simulink model "BD_PAR_AUTO_base_model"  (Simulink 10.3)
settings: Solver=ode1  StartTime=0.0  StopTime=max(cyc_mph(:,1))  FixedStep=1  MaxStep=1  RelTol=1e-3  AbsTol=1e-3
undefined symbols (not defined in the file): acc_dcdc_eff, acc_elec_eff, acc_elec_pwr, acc_mech_eff, acc_mech_pwr, acc_mech_trq, air_cp, amb_tmp, cs_charge_deplete_bool, cs_charge_trq, cs_electric_decel_spd, cs_electric_launch_spd_hi, cs_electric_launch_spd_lo, cs_hi_soc, cs_lo_soc, cs_min_trq_frac, cs_off_trq_frac, cyc_avg_time, cyc_cargo_mass, cyc_elevation_init, cyc_filter_bool, cyc_grade, cyc_mph, enable_sim_stop_distance, enable_sim_stop_max_spd, enable_sim_stop_speed, enable_sim_stop_time, enable_stop, enable_stop_fc, ess_cap_scale, ess_coulombic_eff, ess_init_soc, ess_max_ah_cap, ess_max_volts, ess_min_volts, ess_mod_airflow, ess_mod_cp, ess_mod_init_tmp, ess_module_mass, ess_module_num, ess_on, ess_r_chg, ess_r_dis, ess_res_scale_coef, ess_res_scale_fun, ess_set_tmp, ess_soc, ess_th_calc, ess_th_res_off, ess_th_res_on, ess_tmp, ess_voc, ex_calc, ex_cat_co_frac, ex_cat_ext_cp, ex_cat_ext_emisv, ex_cat_ext_init_tmp, ex_cat_ext_mass, ex_cat_ext_sarea, ex_cat_hc_frac ... (+168)
(part 9 of 15)

== system BD_PAR_AUTO_base_model/electric acc loads <acc>/Electrical Accessory Loads v2 <acc>/backward model/electrical accessories (W)/Electrical Accessories: Time Variable/Elec Aux Loads 14V Pwr/Engine ==
  Average Watts : Constant  Value=vinf.AuxLoads.Engine.AverageWatts
  Memory : Memory
  On : Constant  Value=vinf.AuxLoads.Engine.On
  Product : Product  Inputs=4  InputSameDT=on  RndMeth=Zero  SaturateOnIntegerOverflow=on  OutDataTypeStr=Inherit: Same as first input
  Out1 : Outport
  wires:
  Average Watts/1 -> Product/4
  Product/1 -> Out1/1
  On/1 -> Product/1
  [key_on] -> Product/3
  [engine_on] -> Memory/1
  Memory/1 -> Product/2

== system BD_PAR_AUTO_base_model/electric acc loads <acc>/Electrical Accessory Loads v2 <acc>/backward model/electrical accessories (W)/Electrical Accessories: Time Variable/Elec Aux Loads 14V Pwr/ExternalLights ==
  Average Watts : Constant  Value=vinf.AuxLoads.ExternalLights.AverageWatts
  On : Constant  Value=vinf.AuxLoads.ExternalLights.On
  Product : Product  Inputs=3  InputSameDT=on  RndMeth=Zero  SaturateOnIntegerOverflow=on  OutDataTypeStr=Inherit: Same as first input
  Subsystem : Subsystem  mask{ModelName='ExternalLights'}
      mask prompts: ModelName "Load Name (example: 'Radio')"
  Out1 : Outport
  wires:
  Product/1 -> Out1/1
  Subsystem/1(On/Off Control) -> Product/2
  On/1 -> Product/1
  Average Watts/1 -> Product/3

== system BD_PAR_AUTO_base_model/electric acc loads <acc>/Electrical Accessory Loads v2 <acc>/backward model/electrical accessories (W)/Electrical Accessories: Time Variable/Elec Aux Loads 14V Pwr/FrontHVAC ==
  Average Watts : Constant  Value=vinf.AuxLoads.FrontHVAC.AverageWatts
  On : Constant  Value=vinf.AuxLoads.FrontHVAC.On
  Product : Product  Inputs=3  InputSameDT=on  RndMeth=Zero  SaturateOnIntegerOverflow=on  OutDataTypeStr=Inherit: Same as first input
  Subsystem : Subsystem  mask{ModelName='FrontHVAC'}
      mask prompts: ModelName "Load Name (example: 'Radio')"
  Out1 : Outport
  wires:
  Product/1 -> Out1/1
  Subsystem/1(On/Off Control) -> Product/2
  On/1 -> Product/1
  Average Watts/1 -> Product/3

== system BD_PAR_AUTO_base_model/electric acc loads <acc>/Electrical Accessory Loads v2 <acc>/backward model/electrical accessories (W)/Electrical Accessories: Time Variable/Elec Aux Loads 14V Pwr/FrontWipers ==
  Average Watts : Constant  Value=vinf.AuxLoads.FrontWipers.AverageWatts
  On : Constant  Value=vinf.AuxLoads.FrontWipers.On
  Product : Product  Inputs=3  InputSameDT=on  RndMeth=Zero  SaturateOnIntegerOverflow=on  OutDataTypeStr=Inherit: Same as first input
  Subsystem : Subsystem  mask{ModelName='FrontWipers'}
      mask prompts: ModelName "Load Name (example: 'Radio')"
  Out1 : Outport
  wires:
  Product/1 -> Out1/1
  Subsystem/1(On/Off Control) -> Product/2
  On/1 -> Product/1
  Average Watts/1 -> Product/3

== system BD_PAR_AUTO_base_model/electric acc loads <acc>/Electrical Accessory Loads v2 <acc>/backward model/electrical accessories (W)/Electrical Accessories: Time Variable/Elec Aux Loads 14V Pwr/HeatedSeats ==
  Average Watts : Constant  Value=vinf.AuxLoads.HeatedSeats.AverageWatts
  Num : Constant  Value=vinf.AuxLoads.HeatedSeats.Num
  On : Constant  Value=vinf.AuxLoads.HeatedSeats.On
  Product : Product  Inputs=4  InputSameDT=on  RndMeth=Zero  SaturateOnIntegerOverflow=on  OutDataTypeStr=Inherit: Same as first input
  Subsystem : Subsystem  mask{ModelName='HeatedSeats'}
      mask prompts: ModelName "Load Name (example: 'Radio')"
  Out1 : Outport
  wires:
  Num/1 -> Product/2
  On/1 -> Product/1
  Average Watts/1 -> Product/4
  Product/1 -> Out1/1
  Subsystem/1(On/Off Control) -> Product/3

== system BD_PAR_AUTO_base_model/electric acc loads <acc>/Electrical Accessory Loads v2 <acc>/backward model/electrical accessories (W)/Electrical Accessories: Time Variable/Elec Aux Loads 14V Pwr/Misc ==
  Average Watts : Constant  Value=vinf.AuxLoads.Misc.AverageWatts
  On : Constant  Value=vinf.AuxLoads.Misc.On
  Product : Product  Inputs=3  InputSameDT=on  RndMeth=Zero  SaturateOnIntegerOverflow=on  OutDataTypeStr=Inherit: Same as first input
  Out1 : Outport
  wires:
  Product/1 -> Out1/1
  On/1 -> Product/1
  [key_on] -> Product/2
  Average Watts/1 -> Product/3

== system BD_PAR_AUTO_base_model/electric acc loads <acc>/Electrical Accessory Loads v2 <acc>/backward model/electrical accessories (W)/Electrical Accessories: Time Variable/Elec Aux Loads 14V Pwr/RadiatorCoolingFan ==
  Average Watts : Constant  Value=vinf.AuxLoads.RadiatorCoolingFan.AverageWatts
  On : Constant  Value=vinf.AuxLoads.RadiatorCoolingFan.On
  Product : Product  Inputs=3  InputSameDT=on  RndMeth=Zero  SaturateOnIntegerOverflow=on  OutDataTypeStr=Inherit: Same as first input
  Subsystem : Subsystem  mask{ModelName='RadiatorCoolingFan'}
      mask prompts: ModelName "Load Name (example: 'Radio')"
  Out1 : Outport
  wires:
  Product/1 -> Out1/1
  Subsystem/1(On/Off Control) -> Product/2
  On/1 -> Product/1
  Average Watts/1 -> Product/3

== system BD_PAR_AUTO_base_model/electric acc loads <acc>/Electrical Accessory Loads v2 <acc>/backward model/electrical accessories (W)/Electrical Accessories: Time Variable/Elec Aux Loads 14V Pwr/Radio ==
  Average Watts : Constant  Value=vinf.AuxLoads.Radio.AverageWatts
  Num : Constant  Value=vinf.AuxLoads.Radio.Num
  On : Constant  Value=vinf.AuxLoads.Radio.On
  Product : Product  Inputs=4  InputSameDT=on  RndMeth=Zero  SaturateOnIntegerOverflow=on  OutDataTypeStr=Inherit: Same as first input
  Subsystem : Subsystem  mask{ModelName='Radio'}
      mask prompts: ModelName "Load Name (example: 'Radio')"
  Out1 : Outport
  wires:
  Product/1 -> Out1/1
  Num/1 -> Product/2
  On/1 -> Product/1
  Average Watts/1 -> Product/4
  Subsystem/1(On/Off Control) -> Product/3

== system BD_PAR_AUTO_base_model/electric acc loads <acc>/Electrical Accessory Loads v2 <acc>/backward model/electrical accessories (W)/Electrical Accessories: Time Variable/Elec Aux Loads 14V Pwr/RearDefrost ==
  Average Watts : Constant  Value=vinf.AuxLoads.RearDefrost.AverageWatts
  On : Constant  Value=vinf.AuxLoads.RearDefrost.On
  Product : Product  Inputs=3  InputSameDT=on  RndMeth=Zero  SaturateOnIntegerOverflow=on  OutDataTypeStr=Inherit: Same as first input
  Subsystem : Subsystem  mask{ModelName='RearDefrost'}
      mask prompts: ModelName "Load Name (example: 'Radio')"
  Out1 : Outport
  wires:
  Product/1 -> Out1/1
  On/1 -> Product/1
  Average Watts/1 -> Product/3
  Subsystem/1(On/Off Control) -> Product/2

== system BD_PAR_AUTO_base_model/electric acc loads <acc>/Electrical Accessory Loads v2 <acc>/backward model/electrical accessories (W)/Electrical Accessories: Time Variable/Elec Aux Loads 14V Pwr/RearHVAC ==
  Average Watts : Constant  Value=vinf.AuxLoads.RearHVAC.AverageWatts
  On : Constant  Value=vinf.AuxLoads.RearHVAC.On
  Product : Product  Inputs=3  InputSameDT=on  RndMeth=Zero  SaturateOnIntegerOverflow=on  OutDataTypeStr=Inherit: Same as first input
  Subsystem : Subsystem  mask{ModelName='RearHVAC'}
      mask prompts: ModelName "Load Name (example: 'Radio')"
  Out1 : Outport
  wires:
  Product/1 -> Out1/1
  Subsystem/1(On/Off Control) -> Product/2
  On/1 -> Product/1
  Average Watts/1 -> Product/3

== system BD_PAR_AUTO_base_model/electric acc loads <acc>/Electrical Accessory Loads v2 <acc>/backward model/electrical accessories (W)/Electrical Accessories: Time Variable/Elec Aux Loads 14V Pwr/RearWipers ==
  Average Watts : Constant  Value=vinf.AuxLoads.RearWipers.AverageWatts
  On : Constant  Value=vinf.AuxLoads.RearWipers.On
  Product : Product  Inputs=3  InputSameDT=on  RndMeth=Zero  SaturateOnIntegerOverflow=on  OutDataTypeStr=Inherit: Same as first input
  Subsystem : Subsystem  mask{ModelName='RearWipers'}
      mask prompts: ModelName "Load Name (example: 'Radio')"
  Out1 : Outport
  wires:
  Product/1 -> Out1/1
  Subsystem/1(On/Off Control) -> Product/2
  On/1 -> Product/1
  Average Watts/1 -> Product/3

== system BD_PAR_AUTO_base_model/electric acc loads <acc>/Electrical Accessory Loads v2 <acc>/backward model/electrical accessories (W)/Electrical Accessories: Time Variable/Elec Aux Loads 14V Pwr/Starter ==
  Product1 : Product  InputSameDT=on  RndMeth=Zero  SaturateOnIntegerOverflow=on  OutDataTypeStr=Inherit: Same as first input
  Starter : Subsystem
  starter_load (power) : Constant  Value=vinf.AuxLoads.Starter.AverageWatts
  Out1 : Outport
  wires:
  Product1/1 -> Out1/1
  starter_load (power)/1 -> Product1/2
  Starter/1(Starter_OnOff_Control) -> Product1/1

== system BD_PAR_AUTO_base_model/electric acc loads <acc>/Electrical Accessory Loads v2 <acc>/backward model/electrical accessories (W)/Electrical Accessories: Time Variable/Elec Aux Loads 14V Pwr/TurnSignals ==
  Average Watts : Constant  Value=vinf.AuxLoads.TurnSignals.AverageWatts
  On : Constant  Value=vinf.AuxLoads.TurnSignals.On
  Product : Product  Inputs=3  InputSameDT=on  RndMeth=Zero  SaturateOnIntegerOverflow=on  OutDataTypeStr=Inherit: Same as first input
  Subsystem : Subsystem  mask{ModelName='TurnSignals'}
      mask prompts: ModelName "Load Name (example: 'Radio')"
  Out1 : Outport
  wires:
  Product/1 -> Out1/1
  Subsystem/1(On/Off Control) -> Product/2
  On/1 -> Product/1
  Average Watts/1 -> Product/3

== system BD_PAR_AUTO_base_model/electric acc loads <acc>/Electrical Accessory Loads v2 <acc>/backward model/electrical accessories (W)/Electrical Accessories: Time Variable/Elec Aux Loads HiV Pwr/CurrentLoad1 ==
  Average Watts : Constant  Value=vinf.AuxLoads.CurrentLoad1.AverageWatts
  On : Constant  Value=vinf.AuxLoads.CurrentLoad1.On
  Product : Product  Inputs=3  InputSameDT=on  RndMeth=Zero  SaturateOnIntegerOverflow=on  OutDataTypeStr=Inherit: Same as first input
  Subsystem : Subsystem  mask{ModelName='CurrentLoad1'}
      mask prompts: ModelName "Load Name (example: 'Radio')"
  Out1 : Outport
  wires:
  Average Watts/1 -> Product/3
  On/1 -> Product/1
  Subsystem/1(On/Off Control) -> Product/2
  Product/1 -> Out1/1

== system BD_PAR_AUTO_base_model/electric acc loads <acc>/Electrical Accessory Loads v2 <acc>/backward model/electrical accessories (W)/Electrical Accessories: Time Variable/Elec Aux Loads HiV Pwr/PowerLoad1 ==
  Average Watts : Constant  Value=vinf.AuxLoads.PowerLoad1.AverageWatts
  On : Constant  Value=vinf.AuxLoads.PowerLoad1.On
  Product : Product  Inputs=3  InputSameDT=on  RndMeth=Zero  SaturateOnIntegerOverflow=on  OutDataTypeStr=Inherit: Same as first input
  Subsystem : Subsystem  mask{ModelName='PowerLoad1'}
      mask prompts: ModelName "Load Name (example: 'Radio')"
  Out1 : Outport
  wires:
  Subsystem/1(On/Off Control) -> Product/2
  Average Watts/1 -> Product/3
  On/1 -> Product/1
  Product/1 -> Out1/1

== system BD_PAR_AUTO_base_model/electric acc loads <acc>/Electrical Accessory Loads v2 <acc>/backward model/electrical accessories (W)/Electrical Accessories: Time Variable/Elec Aux Loads HiV Pwr/PowerLoad2 ==
  Average Watts : Constant  Value=vinf.AuxLoads.PowerLoad2.AverageWatts
  On : Constant  Value=vinf.AuxLoads.PowerLoad2.On
  Product : Product  Inputs=3  InputSameDT=on  RndMeth=Zero  SaturateOnIntegerOverflow=on  OutDataTypeStr=Inherit: Same as first input
  Subsystem : Subsystem  mask{ModelName='PowerLoad2'}
      mask prompts: ModelName "Load Name (example: 'Radio')"
  Out1 : Outport
  wires:
  Product/1 -> Out1/1
  On/1 -> Product/1
  Average Watts/1 -> Product/3
  Subsystem/1(On/Off Control) -> Product/2

== system BD_PAR_AUTO_base_model/electric acc loads <acc>/Electrical Accessory Loads v2 <acc>/backward model/electrical accessories (W)/Electrical Accessories: Time Variable/Elec Aux Loads HiV Pwr/PowerLoad3 ==
  Average Watts : Constant  Value=vinf.AuxLoads.PowerLoad3.AverageWatts
  On : Constant  Value=vinf.AuxLoads.PowerLoad3.On
  Product : Product  Inputs=3  InputSameDT=on  RndMeth=Zero  SaturateOnIntegerOverflow=on  OutDataTypeStr=Inherit: Same as first input
  Subsystem : Subsystem  mask{ModelName='PowerLoad3'}
      mask prompts: ModelName "Load Name (example: 'Radio')"
  Out1 : Outport
  wires:
  Subsystem/1(On/Off Control) -> Product/2
  Average Watts/1 -> Product/3
  On/1 -> Product/1
  Product/1 -> Out1/1

== system BD_PAR_AUTO_base_model/electric acc loads <acc>/Electrical Accessory Loads v2 <acc>/backward model/electrical accessories (W)/Electrical Accessories: Time Variable/Elec Aux Loads HiV Pwr/SpeedLoad1 ==
  On : Constant  Value=vinf.AuxLoads.SpeedLoad1.On
  Product : Product  Inputs=3  InputSameDT=on  RndMeth=Zero  SaturateOnIntegerOverflow=on  OutDataTypeStr=Inherit: Same as first input
  Subsystem : Subsystem  mask{ModelName='SpeedLoad1'}
      mask prompts: ModelName "Load Name (example: 'Radio')"
  "rad/s -> rpm1" : Gain  Gain=60/(2*pi)  SaturateOnIntegerOverflow=on  OutDataTypeStr=Inherit: Same as input  ParamDataTypeStr=Inherit: Same as input
  speed (rpm) vs load (watts) : Lookup  InputValues=[vinf.AuxLoads.SpeedLoad1.Data(1,1),vinf.AuxLoads.SpeedLoad1.Data(2,1)]  Table=[vinf.AuxLoads.SpeedLoad1.Data(1,2),vinf.AuxLoads.SpeedLoad1.Data(2,2)]
  Out1 : Outport
  wires:
  "rad/s -> rpm1"/1 -> speed (rpm) vs load (watts)/1
  [w_APU_speed] -> "rad/s -> rpm1"/1
  speed (rpm) vs load (watts)/1 -> Product/3
  On/1 -> Product/1
  Subsystem/1(On/Off Control) -> Product/2
  Product/1 -> Out1/1

== system BD_PAR_AUTO_base_model/electric acc loads <acc>/Electrical Accessory Loads v2 <acc>/backward model/electrical accessories (W)/Electrical Accessories: Time Variable/Elec Aux Loads HiV Pwr/Starter ==
  Product1 : Product  InputSameDT=on  RndMeth=Zero  SaturateOnIntegerOverflow=on  OutDataTypeStr=Inherit: Same as first input
  Starter : Subsystem
  starter_load (power) : Constant  Value=vinf.AuxLoads.Starter.AverageWatts
  Out1 : Outport
  wires:
  Starter/1(Starter_OnOff_Control) -> Product1/1
  starter_load (power)/1 -> Product1/2
  Product1/1 -> Out1/1

== system BD_PAR_AUTO_base_model/mechanical accessory loads <acc>/Mechanical Accessory Loads v2 <acc>/backward model/mechanical accessories (Nm)/Mechanical Accessories: Const Mech Var Elect/Elec Aux Loads 14V Pwr/BrakeLights ==
  Average Watts : Constant  Value=vinf.AuxLoads.BrakeLights.AverageWatts
  Constant : Constant  Value=0
  Constant1 : Constant
  On : Constant  Value=vinf.AuxLoads.BrakeLights.On
  Product : Product  Inputs=4  InputSameDT=on  RndMeth=Zero  SaturateOnIntegerOverflow=on  OutDataTypeStr=Inherit: Same as first input
  Switch : Switch
  Out1 : Outport
  wires:
  Switch/1 -> Product/2
  On/1 -> Product/1
  [key_on] -> Product/3
  Average Watts/1 -> Product/4
  Constant1/1 -> Switch/3
  [F_req] -> Switch/2
  Constant/1 -> Switch/1
  Product/1 -> Out1/1

== system BD_PAR_AUTO_base_model/mechanical accessory loads <acc>/Mechanical Accessory Loads v2 <acc>/backward model/mechanical accessories (Nm)/Mechanical Accessories: Const Mech Var Elect/Elec Aux Loads 14V Pwr/Engine ==
  Average Watts : Constant  Value=vinf.AuxLoads.Engine.AverageWatts
  Memory : Memory
  On : Constant  Value=vinf.AuxLoads.Engine.On
  Product : Product  Inputs=4  InputSameDT=on  RndMeth=Zero  SaturateOnIntegerOverflow=on  OutDataTypeStr=Inherit: Same as first input
  Out1 : Outport
  wires:
  Average Watts/1 -> Product/4
  Product/1 -> Out1/1
  On/1 -> Product/1
  [key_on] -> Product/3
  [engine_on] -> Memory/1
  Memory/1 -> Product/2

== system BD_PAR_AUTO_base_model/mechanical accessory loads <acc>/Mechanical Accessory Loads v2 <acc>/backward model/mechanical accessories (Nm)/Mechanical Accessories: Const Mech Var Elect/Elec Aux Loads 14V Pwr/ExternalLights ==
  Average Watts : Constant  Value=vinf.AuxLoads.ExternalLights.AverageWatts
  On : Constant  Value=vinf.AuxLoads.ExternalLights.On
  Product : Product  Inputs=3  InputSameDT=on  RndMeth=Zero  SaturateOnIntegerOverflow=on  OutDataTypeStr=Inherit: Same as first input
  Subsystem : Subsystem  mask{ModelName='ExternalLights'}
      mask prompts: ModelName "Load Name (example: 'Radio')"
  Out1 : Outport
  wires:
  Product/1 -> Out1/1
  Subsystem/1(On/Off Control) -> Product/2
  On/1 -> Product/1
  Average Watts/1 -> Product/3

== system BD_PAR_AUTO_base_model/mechanical accessory loads <acc>/Mechanical Accessory Loads v2 <acc>/backward model/mechanical accessories (Nm)/Mechanical Accessories: Const Mech Var Elect/Elec Aux Loads 14V Pwr/FrontHVAC ==
  Average Watts : Constant  Value=vinf.AuxLoads.FrontHVAC.AverageWatts
  On : Constant  Value=vinf.AuxLoads.FrontHVAC.On
  Product : Product  Inputs=3  InputSameDT=on  RndMeth=Zero  SaturateOnIntegerOverflow=on  OutDataTypeStr=Inherit: Same as first input
  Subsystem : Subsystem  mask{ModelName='FrontHVAC'}
      mask prompts: ModelName "Load Name (example: 'Radio')"
  Out1 : Outport
  wires:
  Product/1 -> Out1/1
  Subsystem/1(On/Off Control) -> Product/2
  On/1 -> Product/1
  Average Watts/1 -> Product/3

== system BD_PAR_AUTO_base_model/mechanical accessory loads <acc>/Mechanical Accessory Loads v2 <acc>/backward model/mechanical accessories (Nm)/Mechanical Accessories: Const Mech Var Elect/Elec Aux Loads 14V Pwr/FrontWipers ==
  Average Watts : Constant  Value=vinf.AuxLoads.FrontWipers.AverageWatts
  On : Constant  Value=vinf.AuxLoads.FrontWipers.On
  Product : Product  Inputs=3  InputSameDT=on  RndMeth=Zero  SaturateOnIntegerOverflow=on  OutDataTypeStr=Inherit: Same as first input
  Subsystem : Subsystem  mask{ModelName='FrontWipers'}
      mask prompts: ModelName "Load Name (example: 'Radio')"
  Out1 : Outport
  wires:
  Product/1 -> Out1/1
  Subsystem/1(On/Off Control) -> Product/2
  On/1 -> Product/1
  Average Watts/1 -> Product/3

== system BD_PAR_AUTO_base_model/mechanical accessory loads <acc>/Mechanical Accessory Loads v2 <acc>/backward model/mechanical accessories (Nm)/Mechanical Accessories: Const Mech Var Elect/Elec Aux Loads 14V Pwr/HeatedSeats ==
  Average Watts : Constant  Value=vinf.AuxLoads.HeatedSeats.AverageWatts
  Num : Constant  Value=vinf.AuxLoads.HeatedSeats.Num
  On : Constant  Value=vinf.AuxLoads.HeatedSeats.On
  Product : Product  Inputs=4  InputSameDT=on  RndMeth=Zero  SaturateOnIntegerOverflow=on  OutDataTypeStr=Inherit: Same as first input
  Subsystem : Subsystem  mask{ModelName='HeatedSeats'}
      mask prompts: ModelName "Load Name (example: 'Radio')"
  Out1 : Outport
  wires:
  Num/1 -> Product/2
  On/1 -> Product/1
  Average Watts/1 -> Product/4
  Product/1 -> Out1/1
  Subsystem/1(On/Off Control) -> Product/3

== system BD_PAR_AUTO_base_model/mechanical accessory loads <acc>/Mechanical Accessory Loads v2 <acc>/backward model/mechanical accessories (Nm)/Mechanical Accessories: Const Mech Var Elect/Elec Aux Loads 14V Pwr/Misc ==
  Average Watts : Constant  Value=vinf.AuxLoads.Misc.AverageWatts
  On : Constant  Value=vinf.AuxLoads.Misc.On
  Product : Product  Inputs=3  InputSameDT=on  RndMeth=Zero  SaturateOnIntegerOverflow=on  OutDataTypeStr=Inherit: Same as first input
  Out1 : Outport
  wires:
  Product/1 -> Out1/1
  On/1 -> Product/1
  [key_on] -> Product/2
  Average Watts/1 -> Product/3

== system BD_PAR_AUTO_base_model/mechanical accessory loads <acc>/Mechanical Accessory Loads v2 <acc>/backward model/mechanical accessories (Nm)/Mechanical Accessories: Const Mech Var Elect/Elec Aux Loads 14V Pwr/RadiatorCoolingFan ==
  Average Watts : Constant  Value=vinf.AuxLoads.RadiatorCoolingFan.AverageWatts
  On : Constant  Value=vinf.AuxLoads.RadiatorCoolingFan.On
  Product : Product  Inputs=3  InputSameDT=on  RndMeth=Zero  SaturateOnIntegerOverflow=on  OutDataTypeStr=Inherit: Same as first input
  Subsystem : Subsystem  mask{ModelName='RadiatorCoolingFan'}
      mask prompts: ModelName "Load Name (example: 'Radio')"
  Out1 : Outport
  wires:
  Product/1 -> Out1/1
  Subsystem/1(On/Off Control) -> Product/2
  On/1 -> Product/1
  Average Watts/1 -> Product/3

== system BD_PAR_AUTO_base_model/mechanical accessory loads <acc>/Mechanical Accessory Loads v2 <acc>/backward model/mechanical accessories (Nm)/Mechanical Accessories: Const Mech Var Elect/Elec Aux Loads 14V Pwr/Radio ==
  Average Watts : Constant  Value=vinf.AuxLoads.Radio.AverageWatts
  Num : Constant  Value=vinf.AuxLoads.Radio.Num
  On : Constant  Value=vinf.AuxLoads.Radio.On
  Product : Product  Inputs=4  InputSameDT=on  RndMeth=Zero  SaturateOnIntegerOverflow=on  OutDataTypeStr=Inherit: Same as first input
  Subsystem : Subsystem  mask{ModelName='Radio'}
      mask prompts: ModelName "Load Name (example: 'Radio')"
  Out1 : Outport
  wires:
  Product/1 -> Out1/1
  Num/1 -> Product/2
  On/1 -> Product/1
  Average Watts/1 -> Product/4
  Subsystem/1(On/Off Control) -> Product/3

== system BD_PAR_AUTO_base_model/mechanical accessory loads <acc>/Mechanical Accessory Loads v2 <acc>/backward model/mechanical accessories (Nm)/Mechanical Accessories: Const Mech Var Elect/Elec Aux Loads 14V Pwr/RearDefrost ==
  Average Watts : Constant  Value=vinf.AuxLoads.RearDefrost.AverageWatts
  On : Constant  Value=vinf.AuxLoads.RearDefrost.On
  Product : Product  Inputs=3  InputSameDT=on  RndMeth=Zero  SaturateOnIntegerOverflow=on  OutDataTypeStr=Inherit: Same as first input
  Subsystem : Subsystem  mask{ModelName='RearDefrost'}
      mask prompts: ModelName "Load Name (example: 'Radio')"
  Out1 : Outport
  wires:
  Product/1 -> Out1/1
  On/1 -> Product/1
  Average Watts/1 -> Product/3
  Subsystem/1(On/Off Control) -> Product/2

== system BD_PAR_AUTO_base_model/mechanical accessory loads <acc>/Mechanical Accessory Loads v2 <acc>/backward model/mechanical accessories (Nm)/Mechanical Accessories: Const Mech Var Elect/Elec Aux Loads 14V Pwr/RearHVAC ==
  Average Watts : Constant  Value=vinf.AuxLoads.RearHVAC.AverageWatts
  On : Constant  Value=vinf.AuxLoads.RearHVAC.On
  Product : Product  Inputs=3  InputSameDT=on  RndMeth=Zero  SaturateOnIntegerOverflow=on  OutDataTypeStr=Inherit: Same as first input
  Subsystem : Subsystem  mask{ModelName='RearHVAC'}
      mask prompts: ModelName "Load Name (example: 'Radio')"
  Out1 : Outport
  wires:
  Product/1 -> Out1/1
  Subsystem/1(On/Off Control) -> Product/2
  On/1 -> Product/1
  Average Watts/1 -> Product/3

== system BD_PAR_AUTO_base_model/mechanical accessory loads <acc>/Mechanical Accessory Loads v2 <acc>/backward model/mechanical accessories (Nm)/Mechanical Accessories: Const Mech Var Elect/Elec Aux Loads 14V Pwr/RearWipers ==
  Average Watts : Constant  Value=vinf.AuxLoads.RearWipers.AverageWatts
  On : Constant  Value=vinf.AuxLoads.RearWipers.On
  Product : Product  Inputs=3  InputSameDT=on  RndMeth=Zero  SaturateOnIntegerOverflow=on  OutDataTypeStr=Inherit: Same as first input
  Subsystem : Subsystem  mask{ModelName='RearWipers'}
      mask prompts: ModelName "Load Name (example: 'Radio')"
  Out1 : Outport
  wires:
  Product/1 -> Out1/1
  Subsystem/1(On/Off Control) -> Product/2
  On/1 -> Product/1
  Average Watts/1 -> Product/3

== system BD_PAR_AUTO_base_model/mechanical accessory loads <acc>/Mechanical Accessory Loads v2 <acc>/backward model/mechanical accessories (Nm)/Mechanical Accessories: Const Mech Var Elect/Elec Aux Loads 14V Pwr/Starter ==
  Product1 : Product  InputSameDT=on  RndMeth=Zero  SaturateOnIntegerOverflow=on  OutDataTypeStr=Inherit: Same as first input
  Starter : Subsystem
  starter_load (power) : Constant  Value=vinf.AuxLoads.Starter.AverageWatts
  Out1 : Outport
  wires:
  Product1/1 -> Out1/1
  starter_load (power)/1 -> Product1/2
  Starter/1(Starter_OnOff_Control) -> Product1/1

== system BD_PAR_AUTO_base_model/mechanical accessory loads <acc>/Mechanical Accessory Loads v2 <acc>/backward model/mechanical accessories (Nm)/Mechanical Accessories: Const Mech Var Elect/Elec Aux Loads 14V Pwr/TurnSignals ==
  Average Watts : Constant  Value=vinf.AuxLoads.TurnSignals.AverageWatts
  On : Constant  Value=vinf.AuxLoads.TurnSignals.On
  Product : Product  Inputs=3  InputSameDT=on  RndMeth=Zero  SaturateOnIntegerOverflow=on  OutDataTypeStr=Inherit: Same as first input
  Subsystem : Subsystem  mask{ModelName='TurnSignals'}
      mask prompts: ModelName "Load Name (example: 'Radio')"
  Out1 : Outport
  wires:
  Product/1 -> Out1/1
  Subsystem/1(On/Off Control) -> Product/2
  On/1 -> Product/1
  Average Watts/1 -> Product/3

== system BD_PAR_AUTO_base_model/mechanical accessory loads <acc>/Mechanical Accessory Loads v2 <acc>/backward model/mechanical accessories (Nm)/Mechanical Accessories: Const Mech Var Elect/Elec Aux Loads HiV Pwr/CurrentLoad1 ==
  Average Watts : Constant  Value=vinf.AuxLoads.CurrentLoad1.AverageWatts
  On : Constant  Value=vinf.AuxLoads.CurrentLoad1.On
  Product : Product  Inputs=3  InputSameDT=on  RndMeth=Zero  SaturateOnIntegerOverflow=on  OutDataTypeStr=Inherit: Same as first input
  Subsystem : Subsystem  mask{ModelName='CurrentLoad1'}
      mask prompts: ModelName "Load Name (example: 'Radio')"
  Out1 : Outport
  wires:
  Average Watts/1 -> Product/3
  On/1 -> Product/1
  Subsystem/1(On/Off Control) -> Product/2
  Product/1 -> Out1/1

== system BD_PAR_AUTO_base_model/mechanical accessory loads <acc>/Mechanical Accessory Loads v2 <acc>/backward model/mechanical accessories (Nm)/Mechanical Accessories: Const Mech Var Elect/Elec Aux Loads HiV Pwr/PowerLoad1 ==
  Average Watts : Constant  Value=vinf.AuxLoads.PowerLoad1.AverageWatts
  On : Constant  Value=vinf.AuxLoads.PowerLoad1.On
  Product : Product  Inputs=3  InputSameDT=on  RndMeth=Zero  SaturateOnIntegerOverflow=on  OutDataTypeStr=Inherit: Same as first input
  Subsystem : Subsystem  mask{ModelName='PowerLoad1'}
      mask prompts: ModelName "Load Name (example: 'Radio')"
  Out1 : Outport
  wires:
  Subsystem/1(On/Off Control) -> Product/2
  Average Watts/1 -> Product/3
  On/1 -> Product/1
  Product/1 -> Out1/1

== system BD_PAR_AUTO_base_model/mechanical accessory loads <acc>/Mechanical Accessory Loads v2 <acc>/backward model/mechanical accessories (Nm)/Mechanical Accessories: Const Mech Var Elect/Elec Aux Loads HiV Pwr/PowerLoad2 ==
  Average Watts : Constant  Value=vinf.AuxLoads.PowerLoad2.AverageWatts
  On : Constant  Value=vinf.AuxLoads.PowerLoad2.On
  Product : Product  Inputs=3  InputSameDT=on  RndMeth=Zero  SaturateOnIntegerOverflow=on  OutDataTypeStr=Inherit: Same as first input
  Subsystem : Subsystem  mask{ModelName='PowerLoad2'}
      mask prompts: ModelName "Load Name (example: 'Radio')"
  Out1 : Outport
  wires:
  Product/1 -> Out1/1
  On/1 -> Product/1
  Average Watts/1 -> Product/3
  Subsystem/1(On/Off Control) -> Product/2

== system BD_PAR_AUTO_base_model/mechanical accessory loads <acc>/Mechanical Accessory Loads v2 <acc>/backward model/mechanical accessories (Nm)/Mechanical Accessories: Const Mech Var Elect/Elec Aux Loads HiV Pwr/PowerLoad3 ==
  Average Watts : Constant  Value=vinf.AuxLoads.PowerLoad3.AverageWatts
  On : Constant  Value=vinf.AuxLoads.PowerLoad3.On
  Product : Product  Inputs=3  InputSameDT=on  RndMeth=Zero  SaturateOnIntegerOverflow=on  OutDataTypeStr=Inherit: Same as first input
  Subsystem : Subsystem  mask{ModelName='PowerLoad3'}
      mask prompts: ModelName "Load Name (example: 'Radio')"
  Out1 : Outport
  wires:
  Subsystem/1(On/Off Control) -> Product/2
  Average Watts/1 -> Product/3
  On/1 -> Product/1
  Product/1 -> Out1/1

== system BD_PAR_AUTO_base_model/mechanical accessory loads <acc>/Mechanical Accessory Loads v2 <acc>/backward model/mechanical accessories (Nm)/Mechanical Accessories: Const Mech Var Elect/Elec Aux Loads HiV Pwr/SpeedLoad1 ==
  On : Constant  Value=vinf.AuxLoads.SpeedLoad1.On
  Product : Product  Inputs=3  InputSameDT=on  RndMeth=Zero  SaturateOnIntegerOverflow=on  OutDataTypeStr=Inherit: Same as first input
  Subsystem : Subsystem  mask{ModelName='SpeedLoad1'}
      mask prompts: ModelName "Load Name (example: 'Radio')"
  "rad/s -> rpm1" : Gain  Gain=60/(2*pi)  SaturateOnIntegerOverflow=on  OutDataTypeStr=Inherit: Same as input  ParamDataTypeStr=Inherit: Same as input
  speed (rpm) vs load (watts) : Lookup  InputValues=[vinf.AuxLoads.SpeedLoad1.Data(1,1),vinf.AuxLoads.SpeedLoad1.Data(2,1)]  Table=[vinf.AuxLoads.SpeedLoad1.Data(1,2),vinf.AuxLoads.SpeedLoad1.Data(2,2)]
  Out1 : Outport
  wires:
  "rad/s -> rpm1"/1 -> speed (rpm) vs load (watts)/1
  [w_APU_speed] -> "rad/s -> rpm1"/1
  speed (rpm) vs load (watts)/1 -> Product/3
  On/1 -> Product/1
  Subsystem/1(On/Off Control) -> Product/2
  Product/1 -> Out1/1

== system BD_PAR_AUTO_base_model/mechanical accessory loads <acc>/Mechanical Accessory Loads v2 <acc>/backward model/mechanical accessories (Nm)/Mechanical Accessories: Const Mech Var Elect/Elec Aux Loads HiV Pwr/Starter ==
  Product1 : Product  InputSameDT=on  RndMeth=Zero  SaturateOnIntegerOverflow=on  OutDataTypeStr=Inherit: Same as first input
  Starter : Subsystem
  starter_load (power) : Constant  Value=vinf.AuxLoads.Starter.AverageWatts
  Out1 : Outport
  wires:
  Starter/1(Starter_OnOff_Control) -> Product1/1
  starter_load (power)/1 -> Product1/2
  Product1/1 -> Out1/1

== system BD_PAR_AUTO_base_model/<vc> par auto/gearbox control for use w/ AT/Speed Dependent Shifting/shifting/time since last shift/timer/no-lag Reset Integrator/dt ==
  Clock : Clock
  Memory1 : Memory  InitialCondition=-1
  Sum1 : Sum  Inputs=+-  InputSameDT=on  SaturateOnIntegerOverflow=on  OutDataTypeStr=Inherit: Same as first input
  out_1 : Outport  InitialOutput=0
  wires:
  Sum1/1 -> out_1/1
  Memory1/1 -> Sum1/2
  Clock/1 -> Memory1/1, Sum1/1

== system BD_PAR_AUTO_base_model/<vc> par auto/gearbox control for use w/ AT/Speed Dependent Shifting/shifting1/time since last shift/timer/no-lag Reset Integrator/dt ==
  Clock : Clock
  Memory1 : Memory  InitialCondition=-1
  Sum1 : Sum  Inputs=+-  InputSameDT=on  SaturateOnIntegerOverflow=on  OutDataTypeStr=Inherit: Same as first input
  out_1 : Outport  InitialOutput=0
  wires:
  Sum1/1 -> out_1/1
  Memory1/1 -> Sum1/2
  Clock/1 -> Memory1/1, Sum1/1

== system BD_PAR_AUTO_base_model/electric acc loads <acc>/Electrical Accessory Loads v2 <acc>/backward model/electrical accessories (W)/Electrical Accessories: Time Variable/Elec Aux Loads 14V Pwr/ExternalLights/Subsystem ==
  Load On/Off : Switch  Threshold=.5
  On/Off checkbox : Gain  Gain=vinf.AuxLoadsOn  SaturateOnIntegerOverflow=on
  Product : Product  SaturateOnIntegerOverflow=on
  Regular Cycles (1) or Toggle On Off (0) : Constant  Value=strcmp(evalin('base',['vinf.AuxLoads.',ModelName,'.OnOffInfo.Type']),'RegularCycles')
  Subsystem : Subsystem
  Subsystem1 : Subsystem
  On/Off Control : Outport
  wires:
  On/Off checkbox/1 -> On/Off Control/1
  [key_on] -> Product/2
  Load On/Off/1 -> Product/1
  Product/1 -> On/Off checkbox/1
  Regular Cycles (1) or Toggle On Off (0)/1 -> Load On/Off/2
  Subsystem/1(Reg Cycle On/Off) -> Load On/Off/1
  Subsystem1/1(Toggle On/Off) -> Load On/Off/3

== system BD_PAR_AUTO_base_model/electric acc loads <acc>/Electrical Accessory Loads v2 <acc>/backward model/electrical accessories (W)/Electrical Accessories: Time Variable/Elec Aux Loads 14V Pwr/FrontHVAC/Subsystem ==
  Load On/Off : Switch  Threshold=.5
  On/Off checkbox : Gain  Gain=vinf.AuxLoadsOn  SaturateOnIntegerOverflow=on
  Product : Product  SaturateOnIntegerOverflow=on
  Regular Cycles (1) or Toggle On Off (0) : Constant  Value=strcmp(evalin('base',['vinf.AuxLoads.',ModelName,'.OnOffInfo.Type']),'RegularCycles')
  Subsystem : Subsystem
  Subsystem1 : Subsystem
  On/Off Control : Outport
  wires:
  On/Off checkbox/1 -> On/Off Control/1
  [key_on] -> Product/2
  Load On/Off/1 -> Product/1
  Product/1 -> On/Off checkbox/1
  Regular Cycles (1) or Toggle On Off (0)/1 -> Load On/Off/2
  Subsystem/1(Reg Cycle On/Off) -> Load On/Off/1
  Subsystem1/1(Toggle On/Off) -> Load On/Off/3

== system BD_PAR_AUTO_base_model/electric acc loads <acc>/Electrical Accessory Loads v2 <acc>/backward model/electrical accessories (W)/Electrical Accessories: Time Variable/Elec Aux Loads 14V Pwr/FrontWipers/Subsystem ==
  Load On/Off : Switch  Threshold=.5
  On/Off checkbox : Gain  Gain=vinf.AuxLoadsOn  SaturateOnIntegerOverflow=on
  Product : Product  SaturateOnIntegerOverflow=on
  Regular Cycles (1) or Toggle On Off (0) : Constant  Value=strcmp(evalin('base',['vinf.AuxLoads.',ModelName,'.OnOffInfo.Type']),'RegularCycles')
  Subsystem : Subsystem
  Subsystem1 : Subsystem
  On/Off Control : Outport
  wires:
  On/Off checkbox/1 -> On/Off Control/1
  [key_on] -> Product/2
  Load On/Off/1 -> Product/1
  Product/1 -> On/Off checkbox/1
  Regular Cycles (1) or Toggle On Off (0)/1 -> Load On/Off/2
  Subsystem/1(Reg Cycle On/Off) -> Load On/Off/1
  Subsystem1/1(Toggle On/Off) -> Load On/Off/3

== system BD_PAR_AUTO_base_model/electric acc loads <acc>/Electrical Accessory Loads v2 <acc>/backward model/electrical accessories (W)/Electrical Accessories: Time Variable/Elec Aux Loads 14V Pwr/HeatedSeats/Subsystem ==
  Load On/Off : Switch  Threshold=.5
  On/Off checkbox : Gain  Gain=vinf.AuxLoadsOn  SaturateOnIntegerOverflow=on
  Product : Product  SaturateOnIntegerOverflow=on
  Regular Cycles (1) or Toggle On Off (0) : Constant  Value=strcmp(evalin('base',['vinf.AuxLoads.',ModelName,'.OnOffInfo.Type']),'RegularCycles')
  Subsystem : Subsystem
  Subsystem1 : Subsystem
  On/Off Control : Outport
  wires:
  On/Off checkbox/1 -> On/Off Control/1
  [key_on] -> Product/2
  Load On/Off/1 -> Product/1
  Product/1 -> On/Off checkbox/1
  Regular Cycles (1) or Toggle On Off (0)/1 -> Load On/Off/2
  Subsystem/1(Reg Cycle On/Off) -> Load On/Off/1
  Subsystem1/1(Toggle On/Off) -> Load On/Off/3

== system BD_PAR_AUTO_base_model/electric acc loads <acc>/Electrical Accessory Loads v2 <acc>/backward model/electrical accessories (W)/Electrical Accessories: Time Variable/Elec Aux Loads 14V Pwr/RadiatorCoolingFan/Subsystem ==
  Load On/Off : Switch  Threshold=.5
  On/Off checkbox : Gain  Gain=vinf.AuxLoadsOn  SaturateOnIntegerOverflow=on
  Product : Product  SaturateOnIntegerOverflow=on
  Regular Cycles (1) or Toggle On Off (0) : Constant  Value=strcmp(evalin('base',['vinf.AuxLoads.',ModelName,'.OnOffInfo.Type']),'RegularCycles')
  Subsystem : Subsystem
  Subsystem1 : Subsystem
  On/Off Control : Outport
  wires:
  On/Off checkbox/1 -> On/Off Control/1
  [key_on] -> Product/2
  Load On/Off/1 -> Product/1
  Product/1 -> On/Off checkbox/1
  Regular Cycles (1) or Toggle On Off (0)/1 -> Load On/Off/2
  Subsystem/1(Reg Cycle On/Off) -> Load On/Off/1
  Subsystem1/1(Toggle On/Off) -> Load On/Off/3

== system BD_PAR_AUTO_base_model/electric acc loads <acc>/Electrical Accessory Loads v2 <acc>/backward model/electrical accessories (W)/Electrical Accessories: Time Variable/Elec Aux Loads 14V Pwr/Radio/Subsystem ==
  Load On/Off : Switch  Threshold=.5
  On/Off checkbox : Gain  Gain=vinf.AuxLoadsOn  SaturateOnIntegerOverflow=on
  Product : Product  SaturateOnIntegerOverflow=on
  Regular Cycles (1) or Toggle On Off (0) : Constant  Value=strcmp(evalin('base',['vinf.AuxLoads.',ModelName,'.OnOffInfo.Type']),'RegularCycles')
  Subsystem : Subsystem
  Subsystem1 : Subsystem
  On/Off Control : Outport
  wires:
  On/Off checkbox/1 -> On/Off Control/1
  [key_on] -> Product/2
  Load On/Off/1 -> Product/1
  Product/1 -> On/Off checkbox/1
  Regular Cycles (1) or Toggle On Off (0)/1 -> Load On/Off/2
  Subsystem/1(Reg Cycle On/Off) -> Load On/Off/1
  Subsystem1/1(Toggle On/Off) -> Load On/Off/3

== system BD_PAR_AUTO_base_model/electric acc loads <acc>/Electrical Accessory Loads v2 <acc>/backward model/electrical accessories (W)/Electrical Accessories: Time Variable/Elec Aux Loads 14V Pwr/RearDefrost/Subsystem ==
  Load On/Off : Switch  Threshold=.5
  On/Off checkbox : Gain  Gain=vinf.AuxLoadsOn  SaturateOnIntegerOverflow=on
  Product : Product  SaturateOnIntegerOverflow=on
  Regular Cycles (1) or Toggle On Off (0) : Constant  Value=strcmp(evalin('base',['vinf.AuxLoads.',ModelName,'.OnOffInfo.Type']),'RegularCycles')
  Subsystem : Subsystem
  Subsystem1 : Subsystem
  On/Off Control : Outport
  wires:
  On/Off checkbox/1 -> On/Off Control/1
  [key_on] -> Product/2
  Load On/Off/1 -> Product/1
  Product/1 -> On/Off checkbox/1
  Regular Cycles (1) or Toggle On Off (0)/1 -> Load On/Off/2
  Subsystem/1(Reg Cycle On/Off) -> Load On/Off/1
  Subsystem1/1(Toggle On/Off) -> Load On/Off/3

== system BD_PAR_AUTO_base_model/electric acc loads <acc>/Electrical Accessory Loads v2 <acc>/backward model/electrical accessories (W)/Electrical Accessories: Time Variable/Elec Aux Loads 14V Pwr/RearHVAC/Subsystem ==
  Load On/Off : Switch  Threshold=.5
  On/Off checkbox : Gain  Gain=vinf.AuxLoadsOn  SaturateOnIntegerOverflow=on
  Product : Product  SaturateOnIntegerOverflow=on
  Regular Cycles (1) or Toggle On Off (0) : Constant  Value=strcmp(evalin('base',['vinf.AuxLoads.',ModelName,'.OnOffInfo.Type']),'RegularCycles')
  Subsystem : Subsystem
  Subsystem1 : Subsystem
  On/Off Control : Outport
  wires:
  On/Off checkbox/1 -> On/Off Control/1
  [key_on] -> Product/2
  Load On/Off/1 -> Product/1
  Product/1 -> On/Off checkbox/1
  Regular Cycles (1) or Toggle On Off (0)/1 -> Load On/Off/2
  Subsystem/1(Reg Cycle On/Off) -> Load On/Off/1
  Subsystem1/1(Toggle On/Off) -> Load On/Off/3

== system BD_PAR_AUTO_base_model/electric acc loads <acc>/Electrical Accessory Loads v2 <acc>/backward model/electrical accessories (W)/Electrical Accessories: Time Variable/Elec Aux Loads 14V Pwr/RearWipers/Subsystem ==
  Load On/Off : Switch  Threshold=.5
  On/Off checkbox : Gain  Gain=vinf.AuxLoadsOn  SaturateOnIntegerOverflow=on
  Product : Product  SaturateOnIntegerOverflow=on
  Regular Cycles (1) or Toggle On Off (0) : Constant  Value=strcmp(evalin('base',['vinf.AuxLoads.',ModelName,'.OnOffInfo.Type']),'RegularCycles')
  Subsystem : Subsystem
  Subsystem1 : Subsystem
  On/Off Control : Outport
  wires:
  On/Off checkbox/1 -> On/Off Control/1
  [key_on] -> Product/2
  Load On/Off/1 -> Product/1
  Product/1 -> On/Off checkbox/1
  Regular Cycles (1) or Toggle On Off (0)/1 -> Load On/Off/2
  Subsystem/1(Reg Cycle On/Off) -> Load On/Off/1
  Subsystem1/1(Toggle On/Off) -> Load On/Off/3

== system BD_PAR_AUTO_base_model/electric acc loads <acc>/Electrical Accessory Loads v2 <acc>/backward model/electrical accessories (W)/Electrical Accessories: Time Variable/Elec Aux Loads 14V Pwr/Starter/Starter ==
  14 V : Constant  Value=vinf.AuxLoads.Starter.V14
  Hit  Crossing : HitCross  HitCrossingDirection=rising
  Memory : Memory  InitialCondition=fc_on
  On : Constant  Value=vinf.AuxLoads.Starter.On
  Product1 : Product  Inputs=4  SaturateOnIntegerOverflow=on
  Subsystem : Subsystem
  Starter_OnOff_Control : Outport
  wires:
  14 V/1 -> Product1/2
  Subsystem/1(Out1) -> Product1/3
  Product1/1 -> Starter_OnOff_Control/1
  On/1 -> Product1/1
  [key_on] -> Product1/4
  [time] -> Subsystem/2(In2)
  [engine_on] -> Memory/1
  Hit  Crossing/1 -> Subsystem/1(In1)
  Memory/1 -> Hit  Crossing/1

== system BD_PAR_AUTO_base_model/electric acc loads <acc>/Electrical Accessory Loads v2 <acc>/backward model/electrical accessories (W)/Electrical Accessories: Time Variable/Elec Aux Loads 14V Pwr/TurnSignals/Subsystem ==
  Load On/Off : Switch  Threshold=.5
  On/Off checkbox : Gain  Gain=vinf.AuxLoadsOn  SaturateOnIntegerOverflow=on
  Product : Product  SaturateOnIntegerOverflow=on
  Regular Cycles (1) or Toggle On Off (0) : Constant  Value=strcmp(evalin('base',['vinf.AuxLoads.',ModelName,'.OnOffInfo.Type']),'RegularCycles')
  Subsystem : Subsystem
  Subsystem1 : Subsystem
  On/Off Control : Outport
  wires:
  On/Off checkbox/1 -> On/Off Control/1
  [key_on] -> Product/2
  Load On/Off/1 -> Product/1
  Product/1 -> On/Off checkbox/1
  Regular Cycles (1) or Toggle On Off (0)/1 -> Load On/Off/2
  Subsystem/1(Reg Cycle On/Off) -> Load On/Off/1
  Subsystem1/1(Toggle On/Off) -> Load On/Off/3

== system BD_PAR_AUTO_base_model/electric acc loads <acc>/Electrical Accessory Loads v2 <acc>/backward model/electrical accessories (W)/Electrical Accessories: Time Variable/Elec Aux Loads HiV Pwr/CurrentLoad1/Subsystem ==
  Load On/Off : Switch  Threshold=.5
  On/Off checkbox : Gain  Gain=vinf.AuxLoadsOn  SaturateOnIntegerOverflow=on
  Product : Product  SaturateOnIntegerOverflow=on
  Regular Cycles (1) or Toggle On Off (0) : Constant  Value=strcmp(evalin('base',['vinf.AuxLoads.',ModelName,'.OnOffInfo.Type']),'RegularCycles')
  Subsystem : Subsystem
  Subsystem1 : Subsystem
  On/Off Control : Outport
  wires:
  On/Off checkbox/1 -> On/Off Control/1
  [key_on] -> Product/2
  Load On/Off/1 -> Product/1
  Product/1 -> On/Off checkbox/1
  Regular Cycles (1) or Toggle On Off (0)/1 -> Load On/Off/2
  Subsystem/1(Reg Cycle On/Off) -> Load On/Off/1
  Subsystem1/1(Toggle On/Off) -> Load On/Off/3

== system BD_PAR_AUTO_base_model/electric acc loads <acc>/Electrical Accessory Loads v2 <acc>/backward model/electrical accessories (W)/Electrical Accessories: Time Variable/Elec Aux Loads HiV Pwr/PowerLoad1/Subsystem ==
  Load On/Off : Switch  Threshold=.5
  On/Off checkbox : Gain  Gain=vinf.AuxLoadsOn  SaturateOnIntegerOverflow=on
  Product : Product  SaturateOnIntegerOverflow=on
  Regular Cycles (1) or Toggle On Off (0) : Constant  Value=strcmp(evalin('base',['vinf.AuxLoads.',ModelName,'.OnOffInfo.Type']),'RegularCycles')
  Subsystem : Subsystem
  Subsystem1 : Subsystem
  On/Off Control : Outport
  wires:
  On/Off checkbox/1 -> On/Off Control/1
  [key_on] -> Product/2
  Load On/Off/1 -> Product/1
  Product/1 -> On/Off checkbox/1
  Regular Cycles (1) or Toggle On Off (0)/1 -> Load On/Off/2
  Subsystem/1(Reg Cycle On/Off) -> Load On/Off/1
  Subsystem1/1(Toggle On/Off) -> Load On/Off/3

== system BD_PAR_AUTO_base_model/electric acc loads <acc>/Electrical Accessory Loads v2 <acc>/backward model/electrical accessories (W)/Electrical Accessories: Time Variable/Elec Aux Loads HiV Pwr/PowerLoad2/Subsystem ==
  Load On/Off : Switch  Threshold=.5
  On/Off checkbox : Gain  Gain=vinf.AuxLoadsOn  SaturateOnIntegerOverflow=on
  Product : Product  SaturateOnIntegerOverflow=on
  Regular Cycles (1) or Toggle On Off (0) : Constant  Value=strcmp(evalin('base',['vinf.AuxLoads.',ModelName,'.OnOffInfo.Type']),'RegularCycles')
  Subsystem : Subsystem
  Subsystem1 : Subsystem
  On/Off Control : Outport
  wires:
  On/Off checkbox/1 -> On/Off Control/1
  [key_on] -> Product/2
  Load On/Off/1 -> Product/1
  Product/1 -> On/Off checkbox/1
  Regular Cycles (1) or Toggle On Off (0)/1 -> Load On/Off/2
  Subsystem/1(Reg Cycle On/Off) -> Load On/Off/1
  Subsystem1/1(Toggle On/Off) -> Load On/Off/3

== system BD_PAR_AUTO_base_model/electric acc loads <acc>/Electrical Accessory Loads v2 <acc>/backward model/electrical accessories (W)/Electrical Accessories: Time Variable/Elec Aux Loads HiV Pwr/PowerLoad3/Subsystem ==
  Load On/Off : Switch  Threshold=.5
  On/Off checkbox : Gain  Gain=vinf.AuxLoadsOn  SaturateOnIntegerOverflow=on
  Product : Product  SaturateOnIntegerOverflow=on
  Regular Cycles (1) or Toggle On Off (0) : Constant  Value=strcmp(evalin('base',['vinf.AuxLoads.',ModelName,'.OnOffInfo.Type']),'RegularCycles')
  Subsystem : Subsystem
  Subsystem1 : Subsystem
  On/Off Control : Outport
  wires:
  On/Off checkbox/1 -> On/Off Control/1
  [key_on] -> Product/2
  Load On/Off/1 -> Product/1
  Product/1 -> On/Off checkbox/1
  Regular Cycles (1) or Toggle On Off (0)/1 -> Load On/Off/2
  Subsystem/1(Reg Cycle On/Off) -> Load On/Off/1
  Subsystem1/1(Toggle On/Off) -> Load On/Off/3

== system BD_PAR_AUTO_base_model/electric acc loads <acc>/Electrical Accessory Loads v2 <acc>/backward model/electrical accessories (W)/Electrical Accessories: Time Variable/Elec Aux Loads HiV Pwr/SpeedLoad1/Subsystem ==
  Load On/Off : Switch  Threshold=.5
  On/Off checkbox : Gain  Gain=vinf.AuxLoadsOn  SaturateOnIntegerOverflow=on
  Product : Product  SaturateOnIntegerOverflow=on
  Regular Cycles (1) or Toggle On Off (0) : Constant  Value=strcmp(evalin('base',['vinf.AuxLoads.',ModelName,'.OnOffInfo.Type']),'RegularCycles')
  Subsystem : Subsystem
  Subsystem1 : Subsystem
  On/Off Control : Outport
  wires:
  On/Off checkbox/1 -> On/Off Control/1
  [key_on] -> Product/2
  Load On/Off/1 -> Product/1
  Product/1 -> On/Off checkbox/1
  Regular Cycles (1) or Toggle On Off (0)/1 -> Load On/Off/2
  Subsystem/1(Reg Cycle On/Off) -> Load On/Off/1
  Subsystem1/1(Toggle On/Off) -> Load On/Off/3

== system BD_PAR_AUTO_base_model/electric acc loads <acc>/Electrical Accessory Loads v2 <acc>/backward model/electrical accessories (W)/Electrical Accessories: Time Variable/Elec Aux Loads HiV Pwr/Starter/Starter ==
  14 V : Constant  Value=vinf.AuxLoads.Starter.HiV
  Hit  Crossing : HitCross  HitCrossingDirection=rising
  Memory : Memory  InitialCondition=fc_on
  On : Constant  Value=vinf.AuxLoads.Starter.On
  Product1 : Product  Inputs=4  InputSameDT=on  RndMeth=Zero  SaturateOnIntegerOverflow=on  OutDataTypeStr=Inherit: Same as first input
  Subsystem : Subsystem
  Starter_OnOff_Control : Outport
  wires:
  Memory/1 -> Hit  Crossing/1
  Hit  Crossing/1 -> Subsystem/1(In1)
  [engine_on] -> Memory/1
  [time] -> Subsystem/2(In2)
  [key_on] -> Product1/4
  On/1 -> Product1/1
  Product1/1 -> Starter_OnOff_Control/1
  Subsystem/1(Out1) -> Product1/3
  14 V/1 -> Product1/2

== system BD_PAR_AUTO_base_model/mechanical accessory loads <acc>/Mechanical Accessory Loads v2 <acc>/backward model/mechanical accessories (Nm)/Mechanical Accessories: Const Mech Var Elect/Elec Aux Loads 14V Pwr/ExternalLights/Subsystem ==
  Load On/Off : Switch  Threshold=.5
  On/Off checkbox : Gain  Gain=vinf.AuxLoadsOn  SaturateOnIntegerOverflow=on
  Product : Product  SaturateOnIntegerOverflow=on
  Regular Cycles (1) or Toggle On Off (0) : Constant  Value=strcmp(evalin('base',['vinf.AuxLoads.',ModelName,'.OnOffInfo.Type']),'RegularCycles')
  Subsystem : Subsystem
  Subsystem1 : Subsystem
  On/Off Control : Outport
  wires:
  On/Off checkbox/1 -> On/Off Control/1
  [key_on] -> Product/2
  Load On/Off/1 -> Product/1
  Product/1 -> On/Off checkbox/1
  Regular Cycles (1) or Toggle On Off (0)/1 -> Load On/Off/2
  Subsystem/1(Reg Cycle On/Off) -> Load On/Off/1
  Subsystem1/1(Toggle On/Off) -> Load On/Off/3

== system BD_PAR_AUTO_base_model/mechanical accessory loads <acc>/Mechanical Accessory Loads v2 <acc>/backward model/mechanical accessories (Nm)/Mechanical Accessories: Const Mech Var Elect/Elec Aux Loads 14V Pwr/FrontHVAC/Subsystem ==
  Load On/Off : Switch  Threshold=.5
  On/Off checkbox : Gain  Gain=vinf.AuxLoadsOn  SaturateOnIntegerOverflow=on
  Product : Product  SaturateOnIntegerOverflow=on
  Regular Cycles (1) or Toggle On Off (0) : Constant  Value=strcmp(evalin('base',['vinf.AuxLoads.',ModelName,'.OnOffInfo.Type']),'RegularCycles')
  Subsystem : Subsystem
  Subsystem1 : Subsystem
  On/Off Control : Outport
  wires:
  On/Off checkbox/1 -> On/Off Control/1
  [key_on] -> Product/2
  Load On/Off/1 -> Product/1
  Product/1 -> On/Off checkbox/1
  Regular Cycles (1) or Toggle On Off (0)/1 -> Load On/Off/2
  Subsystem/1(Reg Cycle On/Off) -> Load On/Off/1
  Subsystem1/1(Toggle On/Off) -> Load On/Off/3

== system BD_PAR_AUTO_base_model/mechanical accessory loads <acc>/Mechanical Accessory Loads v2 <acc>/backward model/mechanical accessories (Nm)/Mechanical Accessories: Const Mech Var Elect/Elec Aux Loads 14V Pwr/FrontWipers/Subsystem ==
  Load On/Off : Switch  Threshold=.5
  On/Off checkbox : Gain  Gain=vinf.AuxLoadsOn  SaturateOnIntegerOverflow=on
  Product : Product  SaturateOnIntegerOverflow=on
  Regular Cycles (1) or Toggle On Off (0) : Constant  Value=strcmp(evalin('base',['vinf.AuxLoads.',ModelName,'.OnOffInfo.Type']),'RegularCycles')
  Subsystem : Subsystem
  Subsystem1 : Subsystem
  On/Off Control : Outport
  wires:
  On/Off checkbox/1 -> On/Off Control/1
  [key_on] -> Product/2
  Load On/Off/1 -> Product/1
  Product/1 -> On/Off checkbox/1
  Regular Cycles (1) or Toggle On Off (0)/1 -> Load On/Off/2
  Subsystem/1(Reg Cycle On/Off) -> Load On/Off/1
  Subsystem1/1(Toggle On/Off) -> Load On/Off/3

== system BD_PAR_AUTO_base_model/mechanical accessory loads <acc>/Mechanical Accessory Loads v2 <acc>/backward model/mechanical accessories (Nm)/Mechanical Accessories: Const Mech Var Elect/Elec Aux Loads 14V Pwr/HeatedSeats/Subsystem ==
  Load On/Off : Switch  Threshold=.5
  On/Off checkbox : Gain  Gain=vinf.AuxLoadsOn  SaturateOnIntegerOverflow=on
  Product : Product  SaturateOnIntegerOverflow=on
  Regular Cycles (1) or Toggle On Off (0) : Constant  Value=strcmp(evalin('base',['vinf.AuxLoads.',ModelName,'.OnOffInfo.Type']),'RegularCycles')
  Subsystem : Subsystem
  Subsystem1 : Subsystem
  On/Off Control : Outport
  wires:
  On/Off checkbox/1 -> On/Off Control/1
  [key_on] -> Product/2
  Load On/Off/1 -> Product/1
  Product/1 -> On/Off checkbox/1
  Regular Cycles (1) or Toggle On Off (0)/1 -> Load On/Off/2
  Subsystem/1(Reg Cycle On/Off) -> Load On/Off/1
  Subsystem1/1(Toggle On/Off) -> Load On/Off/3
